simulink model "HoornSimulation_fb_lin_2thruster_0rudder"  (R2020b)
settings: Solver=FixedStepAuto  StartTime=0.0  StopTime=4000  FixedStep=0.01  RelTol=1e-3
libraries: pid_lib x2, simulink x1
settings Model: Creator=WANGY17  LastModifiedBy=ASUS
settings SolverCC: AlgebraicLoopSolver=LineSearch
settings DataIOCC: LimitDataPoints=on  SaveFormat=Array  ReturnWorkspaceOutputs=off
settings OptimizationCC: BlockReduction=off  BooleanDataType=off  LifeSpan=inf
settings DebuggingCC: SaveWithParameterizedLinksMsg=none  UnderspecifiedInitializationDetection=Classic  MergeDetectMultiDrivingBlocksExec=none  SignalResolutionControl=TryResolveAllWithWarning  SFUnexpectedBacktrackingDiag=warning  SFNoUnconditionalDefaultTransitionDiag=warning  SFExecutionAtInitializationDiag=none  ArithmeticOperatorsInVariantConditions=warning
settings HardwareCC: ProdBitPerPointer=32  ProdBitPerSizeT=32  ProdBitPerPtrDiffT=32  ProdLargestAtomicFloat=None  ProdIntDivRoundTo=Undefined  ProdEndianess=Unspecified  ProdWordSize=32  ProdHWDeviceType=32-bit Generic  TargetUnknown=on
settings ModelReferenceCC: PropagateSignalLabelsOutOfModel=off
settings SFSimCC: SimUseLocalCustomCode=off  CustomCodeUndefinedFunction=UseInterfaceOnly
settings RTWCC: RTWUseLocalCustomCode=off
settings CodeAppCC: StateflowObjectComments=on
settings GRTTargetCC: TargetLangStandard=C89/C90 (ANSI)
settings ConfigComp: CovMetricSettings=dw  CovSaveCumulativeToWorkspaceVar=on  CovSaveSingleToWorkspaceVar=on  CovExternalEMLEnable=off  CovSFcnEnable=off

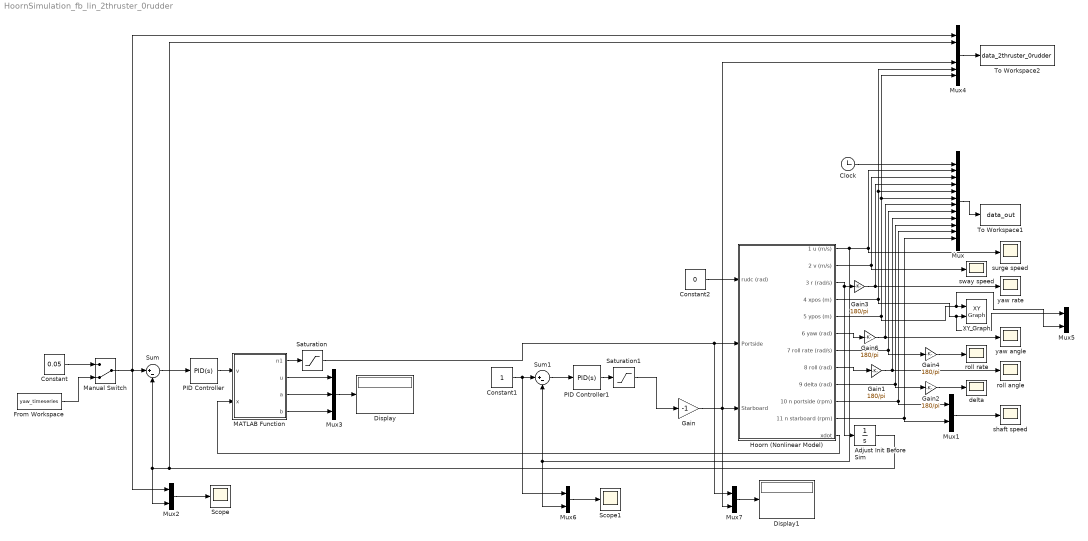
== system HoornSimulation_fb_lin_2thruster_0rudder ==
  Adjust Init Before Sim : Integrator  InitialCondition=3.063052837250049
  Clock : Clock
  Constant : Constant  Value=0.05
  Constant1 : Constant
  Constant2 : Constant  Value=0
  Display : Display
  Display1 : Display
  From Workspace : FromWorkspace  Priority=1  VariableName=yaw_timeseries  Interpolate=off  ZeroCross=off  OutputAfterFinalValue=Holding final value
  Gain : Gain  Gain=-1
  Gain{1..4,6} (5 alike) : Gain  Gain=180/pi
  Hoorn (Nonlinear Model) : Subsystem
  MATLAB Function : MATLAB Function  TreatAsAtomicUnit=on
  Manual Switch : ManualSwitch  CurrentSetting=0
  Mux : Mux  Inputs=12
  Mux{1..2,5..7} (5 alike) : Mux  Inputs=2
  Mux3 : Mux  Inputs=3
  Mux4 : Mux  Inputs=7
  PID Controller : pid_lib/PID Controller  Controller=PID  Form=Parallel  TimeDomain=Continuous-time  UseExternalTs=off  SampleTime=-1  IntegratorMethod=Forward Euler  FilterMethod=Forward Euler  ControllerParametersSource=internal  P=100000  I=0  D=50  UseFilter=on  N=100  TunerSelectOption=Transfer Function Based (PID Tuner App)  InitialConditionSource=internal  InitialConditionForIntegrator=0  InitialConditionForFilter=0  DifferentiatorICPrevScaledInput=0  ExternalReset=none  TrackingMode=off  Kt=1  LimitOutput=off  SatLimitsSource=internal  UpperSaturationLimit=inf  LowerSaturationLimit=-inf  LinearizeAsGain=on  AntiWindupMode=none  Kb=1  POutMin=[]  POutMax=[]  IOutMin=[]  IOutMax=[]  DOutMin=[]  DOutMax=[]  NOutMin=[]  NOutMax=[]  SumOutMin=[]  SumOutMax=[]  SaturationOutMin=[]  SaturationOutMax=[]  PParamMin=[]  PParamMax=[]  IParamMin=[]  IParamMax=[]  DParamMin=[]  DParamMax=[]  NParamMin=[]  NParamMax=[]  KbParamMin=[]  KbParamMax=[]  KtParamMin=[]  KtParamMax=[]  KbOutMin=[]  KbOutMax=[]  KtOutMin=[]  KtOutMax=[]  IntegratorOutMin=[]  IntegratorOutMax=[]  FilterOutMin=[]  FilterOutMax=[]  SumI1OutMin=[]  SumI1OutMax=[]  SumI2OutMin=[]  SumI2OutMax=[]  SumI3OutMin=[]  SumI3OutMax=[]  SumI4OutMin=[]  SumI4OutMax=[]  SumDOutMin=[]  SumDOutMax=[]  DifferentiatorOutMin=[]  DifferentiatorOutMax=[]  FilterDiffOutCoefMin=[]  FilterDiffOutCoefMax=[]  ReciprocalOutMin=[]  ReciprocalOutMax=[]  SumDenOutMin=[]  SumDenOutMax=[]  SumNumOutMin=[]  SumNumOutMax=[]  DivideOutMin=[]  DivideOutMax=[]  UdiffTsProdOutMin=[]  UdiffTsProdOutMax=[]  NTsProdOutMin=[]  NTsProdOutMax=[]  UintegralTsProdOutMin=[]  UintegralTsProdOutMax=[]  UngainTsProdOutMin=[]  UngainTsProdOutMax=[]  IntegratorContinuousStateAttributes=''  IntegratorStateMustResolveToSignalObject=off  IntegratorRTWStateStorageClass=Auto  FilterContinuousStateAttributes=''  FilterStateMustResolveToSignalObject=off  FilterRTWStateStorageClass=Auto  ParallelPVariant=InternalParameters  IdealPVariant=Disabled  IVariant=InternalParameters  DVariant=InternalParameters  IntegratorVariant=Continuous  SatVariant=Disabled  AWVariant=Passthrough  PCopyVariant=Disabled  TRVariant=Disabled  FdbkBlocksVariant=Forward  IdealPFdbkVariant=Disabled  SatFdbkVariant=Disabled  DerivativeFilterVariant=ContFilter  NVariant=InternalParameters  NCopyVariant=Disabled  FilterICVariant=InternalICsFilter  IntegratorICVariant=InternalICs  ExternalResetVariant=Disabled  TRSumVariant=Passthrough  SumFdbkVariant=Disabled  SumVariant=Sum_PID  TsampFilterVariant=InternalTs  TsampNgainVariant=Passthrough  TsampIntegralVariant=Passthrough  ExternalSaturationOutDataTypeStr=Inherit: Same as second input
  PID Controller1 : pid_lib/PID Controller  Controller=PID  Form=Parallel  TimeDomain=Continuous-time  UseExternalTs=off  SampleTime=-1  IntegratorMethod=Forward Euler  FilterMethod=Forward Euler  ControllerParametersSource=internal  P=100000  I=10  D=1  UseFilter=on  N=100  TunerSelectOption=Transfer Function Based (PID Tuner App)  InitialConditionSource=internal  InitialConditionForIntegrator=0  InitialConditionForFilter=0  DifferentiatorICPrevScaledInput=0  ExternalReset=none  TrackingMode=off  Kt=1  LimitOutput=off  SatLimitsSource=internal  UpperSaturationLimit=inf  LowerSaturationLimit=-inf  LinearizeAsGain=on  AntiWindupMode=none  Kb=1  POutMin=[]  POutMax=[]  IOutMin=[]  IOutMax=[]  DOutMin=[]  DOutMax=[]  NOutMin=[]  NOutMax=[]  SumOutMin=[]  SumOutMax=[]  SaturationOutMin=[]  SaturationOutMax=[]  PParamMin=[]  PParamMax=[]  IParamMin=[]  IParamMax=[]  DParamMin=[]  DParamMax=[]  NParamMin=[]  NParamMax=[]  KbParamMin=[]  KbParamMax=[]  KtParamMin=[]  KtParamMax=[]  KbOutMin=[]  KbOutMax=[]  KtOutMin=[]  KtOutMax=[]  IntegratorOutMin=[]  IntegratorOutMax=[]  FilterOutMin=[]  FilterOutMax=[]  SumI1OutMin=[]  SumI1OutMax=[]  SumI2OutMin=[]  SumI2OutMax=[]  SumI3OutMin=[]  SumI3OutMax=[]  SumI4OutMin=[]  SumI4OutMax=[]  SumDOutMin=[]  SumDOutMax=[]  DifferentiatorOutMin=[]  DifferentiatorOutMax=[]  FilterDiffOutCoefMin=[]  FilterDiffOutCoefMax=[]  ReciprocalOutMin=[]  ReciprocalOutMax=[]  SumDenOutMin=[]  SumDenOutMax=[]  SumNumOutMin=[]  SumNumOutMax=[]  DivideOutMin=[]  DivideOutMax=[]  UdiffTsProdOutMin=[]  UdiffTsProdOutMax=[]  NTsProdOutMin=[]  NTsProdOutMax=[]  UintegralTsProdOutMin=[]  UintegralTsProdOutMax=[]  UngainTsProdOutMin=[]  UngainTsProdOutMax=[]  IntegratorContinuousStateAttributes=''  IntegratorStateMustResolveToSignalObject=off  IntegratorRTWStateStorageClass=Auto  FilterContinuousStateAttributes=''  FilterStateMustResolveToSignalObject=off  FilterRTWStateStorageClass=Auto  ParallelPVariant=InternalParameters  IdealPVariant=Disabled  IVariant=InternalParameters  DVariant=InternalParameters  IntegratorVariant=Continuous  SatVariant=Disabled  AWVariant=Passthrough  PCopyVariant=Disabled  TRVariant=Disabled  FdbkBlocksVariant=Forward  IdealPFdbkVariant=Disabled  SatFdbkVariant=Disabled  DerivativeFilterVariant=ContFilter  NVariant=InternalParameters  NCopyVariant=Disabled  FilterICVariant=InternalICsFilter  IntegratorICVariant=InternalICs  ExternalResetVariant=Disabled  TRSumVariant=Passthrough  SumFdbkVariant=Disabled  SumVariant=Sum_PID  TsampFilterVariant=InternalTs  TsampNgainVariant=Passthrough  TsampIntegralVariant=Passthrough  ExternalSaturationOutDataTypeStr=Inherit: Same as second input
  Saturation : Saturate  UpperLimit=1000  LowerLimit=-1000
  Saturation1 : Saturate  UpperLimit=1000  LowerLimit=-1000
  Scope : Scope
  Scope1 : Scope
  Sum : Sum  Inputs=|+-
  Sum1 : Sum  Inputs=|+-
  To Workspace1 : ToWorkspace  VariableName=data_out  SampleTime=-1
      settings: Decimation=2
  To Workspace2 : ToWorkspace  VariableName=data_2thruster_0rudder  SampleTime=-1
      settings: Decimation=2
  XY Graph : simulink/Sinks/XY Graph  xmin=-2000  xmax=2000  ymin=-2000  ymax=2000  st=-1
  delta : Scope
  roll angle : Scope
  roll rate : Scope
  shaft speed : Scope
  surge speed : Scope
  sway speed : Scope
  yaw angle : Scope
  yaw rate : Scope
  wires:
  Hoorn (Nonlinear Model)/4(4 xpos (m)) -> Mux4/6, Mux/5, Mux5/1, XY Graph/2
  Hoorn (Nonlinear Model)/5(5 ypos (m)) -> Mux4/7, Mux/6, Mux5/2, XY Graph/1
  Gain6/1 -> Mux/7, yaw angle/1
  Hoorn (Nonlinear Model)/9(9 delta (rad)) -> Mux/10, Gain2/1
  Gain2/1 -> delta/1
  Hoorn (Nonlinear Model)/8(8 roll (rad)) -> Gain1/1
  Gain1/1 -> Mux/9, roll angle/1
  Hoorn (Nonlinear Model)/7(7 roll rate (rad/s)) -> Mux/8, Gain4/1
  Gain4/1 -> roll rate/1
  Mux/1 -> To Workspace1/1
  Hoorn (Nonlinear Model)/1(1 u (m/s)) -> Mux6/2, Sum1/2, surge speed/1, Mux/2
  Hoorn (Nonlinear Model)/2(2 v (m/s)) -> sway speed/1, Mux/3
  Hoorn (Nonlinear Model)/3(3 r (rad/s)) -> Adjust Init Before Sim/1, Gain3/1
  Hoorn (Nonlinear Model)/10(10 n portside (rpm)) -> Mux/11, Mux1/1
  Hoorn (Nonlinear Model)/6(6 yaw (rad)) -> Gain6/1
  Gain3/1 -> Mux/4, yaw rate/1
  Hoorn (Nonlinear Model)/11(11 n starboard (rpm)) -> Mux/12, Mux1/2
  Mux1/1 -> shaft speed/1
  Clock/1 -> Mux/1
  Sum/1 -> PID Controller/1
  Mux2/1 -> Scope/1
  Hoorn (Nonlinear Model)/12(xdot) -> MATLAB Function/2(x)
  PID Controller/1 -> MATLAB Function/1(v)
  Adjust Init Before Sim/1 -> Mux2/2, Sum/2, Mux4/2
  MATLAB Function/1(n1) -> Saturation/1
  Mux3/1 -> Display/1
  MATLAB Function/2(u) -> Mux3/1
  MATLAB Function/3(a) -> Mux3/2
  MATLAB Function/4(b) -> Mux3/3
  Constant/1 -> Manual Switch/1
  Manual Switch/1 -> Mux2/1, Sum/1, Mux4/1
  Mux4/1 -> To Workspace2/1
  PID Controller1/1 -> Saturation1/1
  Gain/1 -> Mux7/2, Hoorn (Nonlinear Model)/3(Starboard), Mux4/5
  Sum1/1 -> PID Controller1/1
  Constant1/1 -> Mux6/1, Sum1/1
  Mux6/1 -> Scope1/1
  Mux7/1 -> Display1/1
  From Workspace/1 -> Manual Switch/2
  Saturation1/1 -> Gain/1
  Constant2/1 -> Hoorn (Nonlinear Model)/1(rudc (rad))
  Saturation/1 -> Hoorn (Nonlinear Model)/2(Portside), Mux7/1

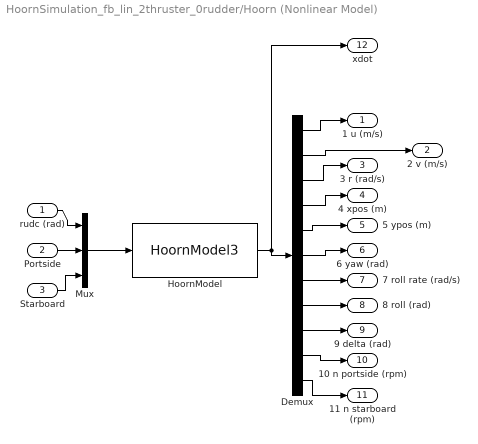
== system HoornSimulation_fb_lin_2thruster_0rudder/Hoorn (Nonlinear Model) ==
  rudc (rad) : Inport
  Portside : Inport  Port=2
  Starboard : Inport  Port=3
  Demux : Demux  Outputs=11
  HoornModel : S-Function  FunctionName=HoornModel3  SFunctionDeploymentMode=off  EnableBusSupport=off
  Mux : Mux  Inputs=3
  1 u (m/s) : Outport
  2 v (m/s) : Outport  Port=2
  3 r (rad/s) : Outport  Port=3
  4 xpos (m) : Outport  Port=4
  5 ypos (m) : Outport  Port=5
  6 yaw (rad) : Outport  Port=6
  7 roll rate (rad/s) : Outport  Port=7
  8 roll (rad) : Outport  Port=8
  9 delta (rad) : Outport  Port=9
  10 n portside (rpm) : Outport  Port=10
  11 n starboard (rpm) : Outport  Port=11
  xdot : Outport  Port=12
  wires:
  Mux/1 -> HoornModel/1
  HoornModel/1 -> xdot/1, Demux/1
  Demux/1 -> 1 u (m/s)/1
  Demux/2 -> 2 v (m/s)/1
  Demux/3 -> 3 r (rad/s)/1
  Demux/4 -> 4 xpos (m)/1
  Demux/5 -> 5 ypos (m)/1
  rudc (rad)/1 -> Mux/1
  Demux/6 -> 6 yaw (rad)/1
  Portside/1 -> Mux/2
  Demux/7 -> 7 roll rate (rad/s)/1
  Demux/8 -> 8 roll (rad)/1
  Demux/9 -> 9 delta (rad)/1
  Demux/10 -> 10 n portside (rpm)/1
  Starboard/1 -> Mux/3
  Demux/11 -> 11 n starboard (rpm)/1

== matlab function HoornSimulation_fb_lin_2thruster_0rudder/MATLAB Function ==
  data: n1 output; v input; x input; u output; a output; b output
function [n1,u,a,b] = fcn(v,x)

% [xdot,U] = container(x,ui) returns the speed U in m/s (optionally) and the 
% time derivative of the state vector: x = [ u v r x y psi p phi delta n ]'  for
% a free running model Hoorn L = 2.47 m, where
%
% u     = surge velocity          (m/s)
% v     = sway velocity           (m/s)
% r     = yaw velocity            (rad/s)
% x     = position in x-direction (m)
% y     = position in y-direction (m)
% psi   = yaw angle               (rad)
% p     = roll velocity           (rad/s)
% phi   = roll angle              (rad)
% delta = actual rudder angle     (rad)
% n1     = propeller 1   (rpm)
% n2     = propeller 2   (rpm)

x1 = x(1);
x2 = x(2);
x3 = x(3);
x4 = x(4);
x5 = x(5);
x6 = x(6);
x7 = x(7);
x8 = x(8);
x9 = x(9);
x10 = x(10);
x11 = x(11);

a = (0.16391*x1^2 + 0.16391*x2^2)*((033257*3.7492e-7)/(x1^2 + x2^2));
b = (0.16391*x1^2 + 0.16391*x2^2)*(- (2.0922*x2)/(x1^2 + x2^2)^(1/2) - (2.8211*x3)/(x1^2 + x2^2)^(1/2) + (0.011225*x8)/(x1^2 + x2^2) + (0.0023799*x7)/(x1^2 + x2^2)^(1/2) + (1.1153*x2^3)/(x1^2 + x2^2)^(3/2) + (6.4192*x3^3)/(x1^2 + x2^2)^(3/2) + (5.6368*x2*x3^2)/(x1^2 + x2^2)^(3/2) - (9.3889*x2^2*x3)/(x1^2 + x2^2)^(3/2) - (4.5351*x2^2*x8)/(x1^2 + x2^2) - (4.8941*x3^2*x8)/(x1^2 + x2^2) - (1.4533*x2*x8^2)/(x1^2 + x2^2)^(1/2) + (1.4854*x3*x8^2)/(x1^2 + x2^2)^(1/2) + (0.13178*x1*x3)/(x1^2 + x2^2));

u = (v - b)/a;
n2 = x11;
l = n2^2+u;
n1 = sign(l)*sqrt(abs(l));
